simulink model "bpsk4"  (R2021b)
settings: Solver=VariableStepAuto  StartTime=0.0  StopTime=10000  RelTol=1e-3
libraries: dsp_blocks x6
settings Model: Creator=aidynardabek  LastModifiedBy=aidynardabek

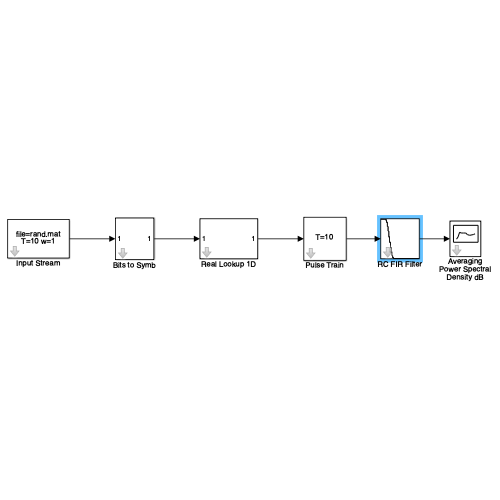
[thumbnail: Simulink's stored preview of the top-level diagram]
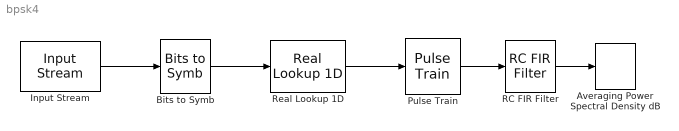
== system bpsk4 ==
  Averaging Power Spectral Density dB : dsp_blocks/Sources//Sinks/Averaging Power Spectral Density dB  npts=128  fftpts=512  HowOften=128  sampleT=1  db_range=40
  Bits to Symb : dsp_blocks/Conversions/Bits to Symb
  Input Stream : dsp_blocks/Sources//Sinks/Input Stream  period=10  width=1  fname=rand.mat
  Pulse Train : dsp_blocks/Conversions/Pulse Train  period=10
  RC FIR Filter : dsp_blocks/Filters/RC FIR Filter  period=10  beta=0.5  root=off  filt_len=128  win_type=off
  Real Lookup 1D : dsp_blocks/Conversions/Real Lookup 1D  table=[-1 1]
  wires:
  Bits to Symb/1 -> Real Lookup 1D/1
  Input Stream/1 -> Bits to Symb/1
  Pulse Train/1 -> RC FIR Filter/1
  Real Lookup 1D/1 -> Pulse Train/1
  RC FIR Filter/1 -> Averaging Power Spectral Density dB/1
